simulink model "FlyingBoard_1engine"  (R2018b)
settings: Solver=FixedStepAuto  StartTime=0.0  StopTime=inf  FixedStep=Ts  RelTol=1e-3  EnableMultiTasking=on
values from neighbouring files (symbols this model uses):
  Ts = 1/100    (= 0.01)    [VTOL_params.m]
undefined symbols (not defined in the file or in its folder): dev, Main, pwm_output0
libraries: pwm_sig_converters x5, px4Sensorslib x3, px4uORBlib x3, simulink x2, px4lib x1, aerolibutil x1, sharedtransform x1
settings Model: SimulationMode=external  ExtModeTrigDuration=10  Creator=Robert  LastModifiedBy=Robert
settings SolverCC: PositivePriorityOrder=on
settings DataIOCC: SaveOutput=off  SignalLogging=off  DSMLogging=off  SaveTime=off
settings OptimizationCC: DefaultUnderspecifiedDataType=single  EnhancedBackFolding=on  PassReuseOutputArgsAs=Individual arguments  MaxStackSize=64  OptimizeBlockOrder=speed  DifferentSizesBufferReuse=on  OptimizationCustomize=off
settings DebuggingCC: ParameterTunabilityLossMsg=error
settings HardwareCC: ProdBitPerPointer=32  ProdBitPerSizeT=32  ProdBitPerPtrDiffT=32  ProdLargestAtomicInteger=Long  ProdLargestAtomicFloat=Double  ProdWordSize=32  ProdLongLongMode=on  ProdHWDeviceType=ARM Compatible->ARM Cortex
settings SFSimCC: MATLABDynamicMemAlloc=off
settings RTWCC: SystemTargetFile=ert.tlc  HardwareBoard=PX4 Pixhawk 1  TLCOptions="-aInlineSetEventsForThisBaseRateFcn=TLC_FALSE -aSuppressMultiTaskScheduler=TLC_FALSE  -aRateBasedStepFcn=0"  TemplateMakefile=ert_default_tmf  GenerateReport=on  Toolchain=GNU Tools for PX4 Autopilots  BuildConfiguration=Faster Runs  IncludeHyperlinkInReport=on  LaunchReport=on  TargetLang=C++  GenerateTraceInfo=on  GenerateTraceReport=on  GenerateTraceReportSl=on  GenerateTraceReportSf=on  GenerateTraceReportEml=on
settings CodeAppCC: ForceParamTrailComments=on  IgnoreCustomStorageClasses=off  OperatorAnnotations=on  SimulinkDataObjDesc=on  SFDataObjDesc=on  InsertBlockDesc=on

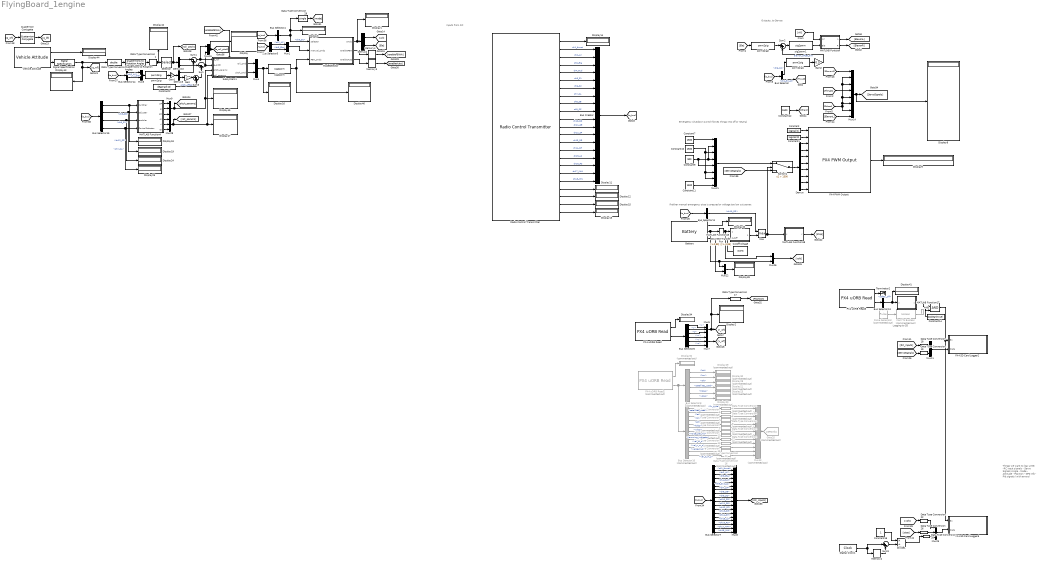
== system FlyingBoard_1engine ==
  note: Emergency shutdown switch forces things into
      | off or neutral
  note: Inputs from RC
  note: Outputs, to Servos
  note: If either manual emergency stop is pressed or voltage too low cut power.
  note: Logging to SD
  note: Things we want to log:
      |
      | uint8
      | -RC input signals
      | - Servo Signals
      |
      | single
      | - Mode
      | - Attitude
      | - Position
      | - GPS info
      | - Pid signals (with errors)
  AND : Logic  IconShape=distinctive  AllPortsSameDT=off  OutDataTypeStr=boolean
  Battery : px4Sensorslib/Battery  voltage=on  current=off  remaining=on  warning=off  timestamp=off  sampleTime=Ts  BlockingMode=off  BlockTimeout=1e-3
      settings: SourceProductName=Embedded Coder Support Package for PX4 Autopilots
  Bus Creator : BusCreator  Inputs=18
  Bus Selector : BusSelector  OutputSignals=ch6_S2,ch1_thrust
  Bus Selector10 : BusSelector  Commented=on  OutputSignals=fix_type,satellites_used,lat,lon,alt,hdop,vdop,noise_per_ms,jamming_indicator,vel_m_s,vel_n_m_s,vel_e_m_s,vel_d_m_s
  Bus Selector11 : BusSelector  OutputSignals=ch10_SD
  Bus Selector13 : BusSelector  OutputSignals=safety_off
  Bus Selector14 : BusSelector  OutputSignals=ch2_Ail,ch3_Ele
  Bus Selector15 : BusSelector  OutputSignals=ch8_SB,ch5_S1,ch12_SF,ch7_SA
  Bus Selector4 : BusSelector  OutputSignals=ch9_SC
  Bus Selector5 : BusSelector  OutputSignals=ch2_Ail,ch3_Ele
  Bus Selector6 : BusSelector  OutputSignals=x,y,z,vx,vy,vz
  Bus Selector7 : BusSelector  OutputSignals=ch1_thrust,ch2_Ail,ch3_Ele,ch4_Rud,ch5_S1,ch6_S2,ch7_SA,ch8_SB,ch9_SC,ch10_SD,ch11_SE,ch12_SF,ch13_SG,ch14_SH,ch15_LS,ch16_RS,ch17_MAX,ch18_MIN
  Bus Selector8 : BusSelector  Commented=on  OutputSignals=lat,lon,alt,satellites_used,hdop,vdop
  Cast To Boolean : DataTypeConversion  Commented=on  OutDataTypeStr=boolean
  Constant : Constant  Value=logical(1)
  Constant1 : Constant  Value=logical(0)
  Constant10 : Constant  Value=1500  OutDataTypeStr=uint16
  Constant11 : Constant  Value=1500  OutDataTypeStr=uint16
  Constant12 : Constant  Value=1500  OutDataTypeStr=uint16  SampleTime=Ts
  Constant14 : Constant  Value=boolean(true)  SampleTime=Ts
  Constant16 : Constant  SampleTime=Ts
  Constant2 : Constant  Value=deg2rad(10)  OutDataTypeStr=single
  Constant7 : Constant  Value=1500  OutDataTypeStr=uint16
  Constant9 : Constant  Value=900  OutDataTypeStr=uint16
  CutoffVoltage : Constant  Value=3.0*3  OutDataTypeStr=single  SampleTime=Ts
  Data Type Conversion : DataTypeConversion  OutDataTypeStr=double
  Data Type Conversion{1,17,22,26,28..29} (6 alike) : DataTypeConversion  OutDataTypeStr=single
  Data Type Conversion{4..16} (13 alike) : DataTypeConversion  Commented=on  OutDataTypeStr=single
  Data Type Conversion18 : DataTypeConversion  OutDataTypeStr=uint16
  Data Type Conversion19 : DataTypeConversion  OutDataTypeStr=uint16
  Demux : Demux  Outputs=8
  Demux10 : Demux  Outputs=2
  Demux2 : Demux  Outputs=2
  Demux3 : Demux  Outputs=2
  Digital Clock1 : DigitalClock  SampleTime=Ts
  Discrete Transfer Fcn : DiscreteTransferFcn  Numerator=[1-0.99]  Denominator=[1 -0.99]  SampleTime=Ts
  Display{,1..3,8..9,11..19,24..25,34,39..46} (26 alike) : Display
      Display9 settings: Format=binary (Stored Integer)
  Display{20..21,23,28..30,32} (7 alike) : Display  Commented=on
  Divide1 : Product  Inputs=*/
  Gain : Gain  Gain=-1
  Gain1 : Gain
  Gain2 : Gain  Gain=0.5
  Goto25 : Goto  Commented=on  GotoTag=GPSinfo
  MATLAB Function : MATLAB Function  TreatAsAtomicUnit=on
  MATLAB Function15 : MATLAB Function  TreatAsAtomicUnit=on
  MATLAB Function17 : MATLAB Function  TreatAsAtomicUnit=on
  MATLAB Function18 : MATLAB Function  TreatAsAtomicUnit=on
  MATLAB Function4 : MATLAB Function  TreatAsAtomicUnit=on
  Max : MinMax  Function=max  Inputs=2  OutDataTypeStr=uint16
  Memory2 : Memory  InheritSampleTime=on
  Memory3 : Memory  InheritSampleTime=on
  Memory4 : Memory  InheritSampleTime=on
  ModeSelector : MATLAB Function  TreatAsAtomicUnit=on
  Mux{1,3..4,11,15,22,26} (7 alike) : Mux  Inputs=2
  Mux13 : Mux  Commented=on  Inputs=13
  Mux14 : Mux  Inputs=8
  Mux21 : Mux  Inputs=8
  Mux{5,7,9,25,28} (5 alike) : Mux  Inputs=3
  Mux8 : Mux  Inputs=18
  PX4 PWM Output : px4lib/PX4 PWM Output  pwmDevice=Main (/dev/pwm_output0)  pwmChannel1_=on  pwmChannel2_=on  pwmChannel3_=on  pwmChannel4_=on  pwmChannel5_=on  pwmChannel6_=on  pwmChannel7_=on  pwmChannel8_=on  forceTerminateFailsafe=off  outputErrorStatus=on
      settings: SourceProductName=Embedded Coder Support Package for PX4 Autopilots
  PX4 SD Card Logger2 : Subsystem  mask(PX4 SD Card Logger){logfile=/fs/microsd/log, logfilename=rc_and_servosignals, cacheflag=off, numRecs=250*60*60}
      mask prompts: logfile "Log Folder"; logfilename "Log File Name"; cacheflag "Cache in Memory"; numRecs "Maximum Record Count"
      mask help:
      | Log data to a specified file on the SD card
      |
      | The block accepts two inputs, enable and data. The incoming data is logged into the SD card when the enable signal is high and the number of data points logged is less than the Maximum Record Count specified.
      |
      | The specified folder should be present in the SD card for logging.
      |
      | If Cache in Memory is unchecked, the data is written to the SD card at every timestep.  If Cache in Memory is checked, data is cached in the memory and is written to SD card only when enable goes low or when the number of data points logged reaches the Maximum Record Count specified.
      mask init:
      | logname=uint8([logfile,'/',logfilename]);
      mask Help: eval('codertarget.internal.helpView(''px4'',''px4sdcardexample'')');
      mask Display:
      | fprintf([get_param(gcb,'logfile'),'/',get_param(gcb,'logfilename')])
      | port_label('input',1,'en')
      | port_label('input',2,'data')
  PX4 SD Card Logger6 : Subsystem  mask(PX4 SD Card Logger){logfile=/fs/microsd/log, logfilename=volt_stop, cacheflag=off, numRecs=250*60*60}
      mask prompts: logfile "Log Folder"; logfilename "Log File Name"; cacheflag "Cache in Memory"; numRecs "Maximum Record Count"
      mask help:
      | Log data to a specified file on the SD card
      |
      | The block accepts two inputs, enable and data. The incoming data is logged into the SD card when the enable signal is high and the number of data points logged is less than the Maximum Record Count specified.
      |
      | The specified folder should be present in the SD card for logging.
      |
      | If Cache in Memory is unchecked, the data is written to the SD card at every timestep.  If Cache in Memory is checked, data is cached in the memory and is written to SD card only when enable goes low or when the number of data points logged reaches the Maximum Record Count specified.
      mask init:
      | logname=uint8([logfile,'/',logfilename]);
      mask Help: eval('codertarget.internal.helpView(''px4'',''px4sdcardexample'')');
      mask Display:
      | fprintf([get_param(gcb,'logfile'),'/',get_param(gcb,'logfilename')])
      | port_label('input',1,'en')
      | port_label('input',2,'data')
  PX4 uORB Read : px4uORBlib/PX4 uORB Read  uORBTopic=vehicle_local_position  sampleTime=Ts  BlockingMode=off  BlockTimeout=1e-3
      settings: SourceProductName=Embedded Coder Support Package for PX4 Autopilots
  PX4 uORB Read2 : px4uORBlib/PX4 uORB Read  Commented=on  uORBTopic=vehicle_gps_position  sampleTime=0.004  BlockingMode=off  BlockTimeout=1e-3
      settings: SourceProductName=Embedded Coder Support Package for PX4 Autopilots
  PX4 uORB Read3 : px4uORBlib/PX4 uORB Read  uORBTopic=safety  sampleTime=Ts  BlockingMode=off  BlockTimeout=1e-3
      settings: SourceProductName=Embedded Coder Support Package for PX4 Autopilots
  Pulse Generator : DiscretePulseGenerator  Commented=on  SampleTime=Ts
  Quaternion Conjugate : aerolibutil/Quaternion Conjugate
      settings: SourceProductName=Aerospace Blockset  SourceProductBaseCode=AE
  Quaternions to Rotation Angles : sharedtransform/Quaternions to Rotation Angles  rotationOrder=ZYX  aMode=aMode
      settings: SourceProductBaseCode=AE
  Radio Control Transmitter : px4Sensorslib/Radio Control Transmitter  channel1=on  channel2=on  channel3=on  channel4=on  channel5=on  channel6=on  channel7=on  channel8=on  channel9=on  channel10=on  channel11=on  channel12=on  channel13=on  channel14=on  channel15=on  channel16=on  channel17=on  channel18=on  channel_count=on  rssi=on  rc_input_source=on  timestamp_last_signal=on  time_stamp=off  sampleTime=Ts  BlockingMode=off  BlockTimeout=5
      settings: SourceProductName=Embedded Coder Support Package for PX4 Autopilots
  Selector : Selector  InputPortWidth=3  IndexOptions=Index vector (dialog)  Indices=[3 2]  OutputSizes=1
  Signal Specification : SignalSpecification  OutDataTypeStr=single
  Subsystem1 : Subsystem
  Sum : Sum  Inputs=|-+
  Sum1 : Sum  Inputs=|-+
  Sum2 : Sum  Inputs=|++
  Sum3 : Sum  Inputs=|++
  Sum9 : Sum  Inputs=|+-
  Switch1 : Switch  Criteria=u2 > Threshold  Threshold=1300
  Terminator2 : Terminator
  Vehicle Attitude : px4Sensorslib/Vehicle Attitude  rollRate=off  pitchRate=off  yawRate=off  quaternion=on  uorbTimeStamp=off  BlockingMode=off  BlockTimeout=0.001  sampleTime=Ts
      settings: SourceProductName=Embedded Coder Support Package for PX4 Autopilots
  pwm2sig : pwm_sig_converters/pwm2sig  SystemSampleTime=-1
  pwm2sig1 : pwm_sig_converters/pwm2sig  SystemSampleTime=-1
  pwm2sig2 : pwm_sig_converters/pwm2sig  SystemSampleTime=-1
  sig2pwm : pwm_sig_converters/sig2pwm  SystemSampleTime=-1
  sig2pwm1 : pwm_sig_converters/sig2pwm  SystemSampleTime=-1
  wires:
  Bus Selector7/10 -> Mux8/10  "<ch10_SD>"
  Battery/3 -> Mux22/2
  [rc_bus] -> Bus Selector11/1
  Switch1/1 -> Demux/1
  Battery/2 -> Discrete Transfer Fcn/1, Mux26/2, Mux22/1
  Demux/8 -> PX4 PWM Output/10
  Data Type Conversion8/1 -> Mux13/5
  Constant11/1 -> Mux21/8
  Radio Control Transmitter/16 -> Bus Creator/15  "ch15_LS"
  Constant7/1 -> Mux21/1
  Demux/1 -> PX4 PWM Output/3
  Constant9/1 -> Mux21/2, Mux21/4, Mux21/5
  Bus Selector7/2 -> Mux8/2  "<ch2_Ail>"
  Radio Control Transmitter/8 -> Bus Creator/7  "ch7_SA"
  [ServoSignals] -> Switch1/3
  Bus Selector10/2 -> Data Type Conversion5/1  "<satellites_used>"
  Max/1 -> MATLAB Function18/1(u), Switch1/2
  Bus Selector7/3 -> Mux8/3  "<ch3_Ele>"
  Bus Selector10/6 -> Data Type Conversion9/1  "<hdop>"
  Data Type Conversion6/1 -> Mux13/3
  Constant10/1 -> Mux21/7, Mux21/6, Mux21/3
  Bus Selector6/5 -> Mux7/2  "<vy>"
  MATLAB Function15/1(stopsig) -> Max/2
  Radio Control Transmitter/19 -> Bus Creator/18  "ch18_MIN"
  Data Type Conversion9/1 -> Mux13/6
  Bus Selector8/4 -> Display21/1  "<satellites_used>"
  Bus Selector10/10 -> Data Type Conversion13/1  "<vel_m_s>"
  Bus Selector6/1 -> Mux5/1  "<x>"
  PX4 PWM Output/1 -> Display9/1
  Mux22/1 -> Display39/1
  Bus Selector11/1 -> Max/1  "<ch10_SD>"
  Radio Control Transmitter/21 -> Display12/1
  Demux/4 -> PX4 PWM Output/6
  Data Type Conversion7/1 -> Mux13/4
  Bus Selector10/9 -> Data Type Conversion12/1  "<jamming_indicator>"
  Demux/3 -> PX4 PWM Output/5
  Bus Selector8/1 -> Display29/1  "<lat>"
  Mux21/1 -> Switch1/1
  Bus Selector7/8 -> Mux8/8  "<ch8_SB>"
  Data Type Conversion16/1 -> Mux13/13
  Radio Control Transmitter/6 -> Bus Creator/5  "ch5_S1"
  [ElevonR] -> Mux14/1
  Bus Selector10/11 -> Data Type Conversion14/1  "<vel_n_m_s>"
  Bus Selector6/4 -> Mux7/1  "<vx>"
  Bus Selector10/8 -> Data Type Conversion11/1  "<noise_per_ms>"
  Data Type Conversion14/1 -> Mux13/11
  Bus Selector10/12 -> Data Type Conversion15/1  "<vel_e_m_s>"
  Bus Selector7/15 -> Mux8/15  "<ch15_LS>"
  Data Type Conversion12/1 -> Mux13/9
  Data Type Conversion13/1 -> Mux13/10
  Bus Selector7/9 -> Mux8/9  "<ch9_SC>"
  Data Type Conversion10/1 -> Mux13/7
  Data Type Conversion5/1 -> Mux13/2
  Demux/6 -> PX4 PWM Output/8
  Demux/7 -> PX4 PWM Output/9
  Mux7/1 -> [v_wf]
  Mux14/1 -> Display8/1, [ServoSignals]
  Bus Selector7/12 -> Mux8/12  "<ch12_SF>"
  Radio Control Transmitter/3 -> Bus Creator/2  "ch2_Ail"
  Bus Selector7/14 -> Mux8/14  "<ch14_SH>"
  Bus Selector7/11 -> Mux8/11  "<ch11_SE>"
  Radio Control Transmitter/23 -> Display13/1
  Bus Selector10/1 -> Data Type Conversion4/1  "<fix_type>"
  [rc_bus] -> Bus Selector7/1
  Bus Selector7/6 -> Mux8/6  "<ch6_S2>"
  Bus Selector10/13 -> Data Type Conversion16/1  "<vel_d_m_s>"
  Bus Selector7/7 -> Mux8/7  "<ch7_SA>"
  Bus Selector7/18 -> Mux8/18  "<ch18_MIN>"
  Data Type Conversion17/1 -> [Position]
  Bus Selector7/4 -> Mux8/4  "<ch4_Rud>"
  Bus Selector7/17 -> Mux8/17  "<ch17_MAX>"
  Radio Control Transmitter/17 -> Bus Creator/16  "ch16_RS"
  Demux/2 -> PX4 PWM Output/4
  Bus Selector7/16 -> Mux8/16  "<ch16_RS>"
  Data Type Conversion11/1 -> Mux13/8
  Radio Control Transmitter/11 -> Bus Creator/10  "ch10_SD"
  Radio Control Transmitter/20 -> Display11/1
  [ElevonL] -> Mux14/8
  PX4 uORB Read/1 -> Display34/1
  [Thrust] -> Mux14/4
  Bus Selector10/4 -> Data Type Conversion7/1  "<lon>"
  Data Type Conversion4/1 -> Mux13/1
  Radio Control Transmitter/14 -> Bus Creator/13  "ch13_SG"
  Bus Selector6/3 -> Mux5/3  "<z>"
  Bus Selector8/2 -> Display30/1  "<lon>"
  PX4 uORB Read/2 -> Bus Selector6/1
  CutoffVoltage/1 -> MATLAB Function15/2(cutoff)
  Radio Control Transmitter/22 -> Display15/1
  Radio Control Transmitter/10 -> Bus Creator/9  "ch9_SC"
  Radio Control Transmitter/15 -> Bus Creator/14  "ch14_SH"
  Radio Control Transmitter/13 -> Bus Creator/12  "ch12_SF"
  Bus Selector7/1 -> Mux8/1  "<ch1_thrust>"
  Radio Control Transmitter/18 -> Bus Creator/17  "ch17_MAX"
  Battery/1 -> Display40/1
  Mux8/1 -> [RC_inputs]
  Bus Selector10/3 -> Data Type Conversion6/1  "<lat>"
  PX4 uORB Read2/1 -> Display32/1
  Radio Control Transmitter/4 -> Bus Creator/3  "ch3_Ele"
  Constant1/1 -> PX4 PWM Output/2
  Bus Creator/1 -> [rc_bus]
  Bus Selector6/6 -> Mux7/3  "<vz>"
  Radio Control Transmitter/5 -> Bus Creator/4  "ch4_Rud"
  Constant/1 -> PX4 PWM Output/1
  Constant12/1 -> [Others]
  Bus Selector7/5 -> Mux8/5  "<ch5_S1>"
  Radio Control Transmitter/1 -> Display14/1
  Radio Control Transmitter/9 -> Bus Creator/8  "ch8_SB"
  PX4 uORB Read2/2 -> Bus Selector10/1, Bus Selector8/1
  Radio Control Transmitter/2 -> Bus Creator/1  "ch1_thrust"
  Bus Selector10/5 -> Data Type Conversion8/1  "<alt>"
  Bus Selector6/2 -> Mux5/2  "<y>"
  Mux13/1 -> Goto25/1
  Radio Control Transmitter/12 -> Bus Creator/11  "ch11_SE"
  Bus Selector7/13 -> Mux8/13  "<ch13_SG>"
  Mux5/1 -> Data Type Conversion17/1, Display2/1, [r_wf]
  Radio Control Transmitter/7 -> Bus Creator/6  "ch6_S2"
  Bus Selector10/7 -> Data Type Conversion10/1  "<vdop>"
  Data Type Conversion15/1 -> Mux13/12
  Bus Selector8/5 -> Display23/1  "<hdop>"
  Demux/5 -> PX4 PWM Output/7
  Bus Selector8/3 -> Display28/1  "<alt>"
  Bus Selector8/6 -> Display20/1  "<vdop>"
  PX4 uORB Read3/2 -> Bus Selector13/1
  Bus Selector13/1 -> MATLAB Function17/1(u), Display41/1  "<safety_off>"
  MATLAB Function17/1(y) -> AND/1
  [RC_inputs] -> Data Type Conversion18/1
  [ServoSignals] -> Data Type Conversion19/1
  Data Type Conversion18/1 -> Mux11/1
  Data Type Conversion19/1 -> Mux11/2
  Mux11/1 -> PX4 SD Card Logger2/2(Data)
  Pulse Generator/1 -> Cast To Boolean/1
  Cast To Boolean/1 -> ?
  Mux25/1 -> PX4 SD Card Logger6/2(Data)
  Data Type Conversion26/1 -> Mux25/2
  AND/1 -> PX4 SD Card Logger6/1(En), PX4 SD Card Logger2/1(En)
  [stop] -> Data Type Conversion26/1
  Data Type Conversion22/1 -> Mux25/1
  [volt] -> Data Type Conversion22/1
  MATLAB Function18/1(y) -> [stop]
  PX4 uORB Read3/1 -> Terminator2/1
  Discrete Transfer Fcn/1 -> MATLAB Function15/1(voltage), Mux26/1
  Mux26/1 -> [volt]
  Constant14/1 -> AND/2
  Divide1/1 -> Data Type Conversion28/1
  Sum9/1 -> Divide1/2
  Constant16/1 -> Divide1/1
  Memory2/1 -> Sum9/2
  Digital Clock1/1 -> Sum9/1, Memory2/1
  Data Type Conversion28/1 -> Mux25/3
  ModeSelector/2(enableFBW) -> Memory4/1
  Memory4/1 -> [enableFBWA]
  Demux10/2 -> Sum/1
  Subsystem1/2(pitch_cmd) -> Mux4/2
  Data Type Conversion29/1 -> [mode]
  Bus Selector15/4 -> Display25/1, MATLAB Function4/4(ControlSelector)  "<ch7_SA>"
  sig2pwm/1 -> ModeSelector/3(FBW_cmds), Display46/1
  Sum1/1 -> Mux15/1, Subsystem1/1(e_roll)
  Demux2/2 -> [Ele]
  Mux15/1 -> Display/1, [e_roll_pitch]
  MATLAB Function4/4(rP) -> Mux28/1
  [q_wf] -> Quaternion Conjugate/1
  ModeSelector/1(cmds) -> Display1/1, Demux2/1
  Memory3/1 -> [enableAuto]
  Bus Selector15/1 -> Display18/1, MATLAB Function4/1(switcher)  "<ch8_SB>"
  pwm2sig/1 -> Gain1/1
  ModeSelector/3(enableAuto) -> Memory3/1
  Mux9/1 -> [pitch_params], Subsystem1/3(pitch_params), Display45/1
  [enableFBWA] -> Subsystem1/Enable
  [rc_bus] -> Bus Selector4/1
  Signal Specification/1 -> [q_wf], Display43/1, Data Type Conversion/1
  MATLAB Function4/3(pD) -> Mux9/3
  Demux10/1 -> Sum1/1
  [rc_bus] -> Bus Selector5/1
  Mux4/1 -> sig2pwm/1, Display16/1
  Mux3/1 -> pwm2sig/1
  [rc_bus] -> Bus Selector15/1
  Bus Selector4/1 -> ModeSelector/1(selector), Display3/1, Data Type Conversion29/1  "<ch9_SC>"
  Data Type Conversion/1 -> Quaternions to Rotation Angles/1
  MATLAB Function4/2(pI) -> Mux9/2
  Demux3/2 -> Gain/1
  [rc_bus] -> Bus Selector14/1
  Mux1/1 -> ModeSelector/2(manual_cmds)
  Data Type Conversion1/1 -> Display42/1, Selector/1
  Bus Selector15/3 -> Display24/1, MATLAB Function4/3(enabler)  "<ch12_SF>"
  Demux2/1 -> [Ail]
  Sum/1 -> Subsystem1/2(e_pitch), Mux15/2
  MATLAB Function4/5(rI) -> Mux28/2
  Bus Selector14/2 -> Mux3/2  "<ch3_Ele>"
  Quaternion Conjugate/1 -> [q_bf]
  MATLAB Function4/6(rD) -> Mux28/3
  Quaternions to Rotation Angles/1 -> Data Type Conversion1/1
  Mux28/1 -> [roll_params], Subsystem1/4(roll_params), Display17/1
  Bus Selector5/2 -> Mux1/2  "<ch3_Ele>"
  Vehicle Attitude/2 -> Signal Specification/1
  Vehicle Attitude/1 -> Display44/1
  Bus Selector14/1 -> Mux3/1  "<ch2_Ail>"
  Bus Selector5/1 -> Mux1/1  "<ch2_Ail>"
  Subsystem1/1(roll_cmd) -> Mux4/1
  Bus Selector15/2 -> Display19/1, MATLAB Function4/2(adjuster)  "<ch5_S1>"
  MATLAB Function4/1(pP) -> Mux9/1
  Selector/1 -> [roll_pitch], Demux10/1
  [Others] -> Mux14/5, Mux14/2, Mux14/3, Mux14/6, Mux14/7
  [Ail] -> MATLAB Function/1(Ail)
  Sum2/1 -> sig2pwm1/1
  MATLAB Function/2(R) -> [ElevonR]
  MATLAB Function/1(L) -> [ElevonL]
  [rc_bus] -> Bus Selector/1
  Bus Selector/2 -> [Thrust]  "<ch1_thrust>"
  Sum3/1 -> Sum/2
  Demux3/1 -> Sum1/2
  Gain1/1 -> Demux3/1
  [Ele] -> pwm2sig2/1
  Bus Selector/1 -> pwm2sig1/1  "<ch6_S2>"
  pwm2sig1/1 -> Gain2/1
  Gain2/1 -> Sum2/2  "elevon_offset_trim"
  pwm2sig2/1 -> Sum2/1
  sig2pwm1/1 -> MATLAB Function/2(Ele)
  Gain/1 -> Sum3/1
  Constant2/1 -> Sum3/2  "pitch_offset"

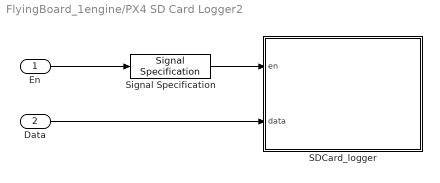
== system FlyingBoard_1engine/PX4 SD Card Logger2 ==
  En : Inport
  Data : Inport  Port=2
  SDCard_logger : MATLAB Function  TreatAsAtomicUnit=on
  Signal Specification : SignalSpecification  OutDataTypeStr=boolean
  wires:
  Signal Specification/1 -> SDCard_logger/1(en)
  En/1 -> Signal Specification/1
  Data/1 -> SDCard_logger/2(data)

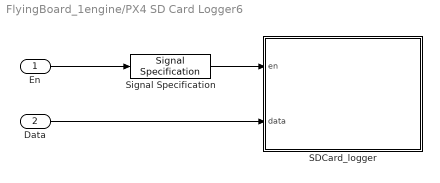
== system FlyingBoard_1engine/PX4 SD Card Logger6 ==
  En : Inport
  Data : Inport  Port=2
  SDCard_logger : MATLAB Function  TreatAsAtomicUnit=on
  Signal Specification : SignalSpecification  OutDataTypeStr=boolean
  wires:
  Signal Specification/1 -> SDCard_logger/1(en)
  En/1 -> Signal Specification/1
  Data/1 -> SDCard_logger/2(data)

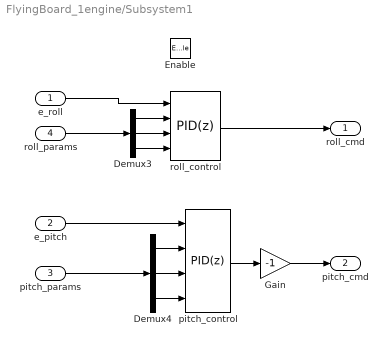
== system FlyingBoard_1engine/Subsystem1 ==
  e_roll : Inport
  e_pitch : Inport  Port=2
  pitch_params : Inport  Port=3
  roll_params : Inport  Port=4
  Enable : EnablePort
  Demux3 : Demux  Outputs=3
  Demux4 : Demux  Outputs=3
  Gain : Gain  Gain=-1
  pitch_control : simulink/Continuous/PID Controller  Controller=PID  Form=Parallel  TimeDomain=Discrete-time  SampleTime=Ts  IntegratorMethod=Backward Euler  FilterMethod=Forward Euler  ControllerParametersSource=external  P=1  I=0  D=0  UseFilter=off  N=100  TunerSelectOption=Transfer Function Based (PID Tuner App)  InitialConditionSource=internal  InitialConditionForIntegrator=0  InitialConditionForFilter=0  DifferentiatorICPrevScaledInput=0  ExternalReset=none  TrackingMode=off  Kt=1  LimitOutput=on  UpperSaturationLimit=1  LowerSaturationLimit=-1  LinearizeAsGain=off  AntiWindupMode=clamping  Kb=1  PGainOutDataTypeStr=single  PProdOutDataTypeStr=single  POutMin=[]  POutMax=[]  IGainOutDataTypeStr=single  IProdOutDataTypeStr=single  IOutMin=[]  IOutMax=[]  DGainOutDataTypeStr=single  DProdOutDataTypeStr=single  DOutMin=[]  DOutMax=[]  NOutMin=[]  NOutMax=[]  SumOutDataTypeStr=single  SumOutMin=[]  SumOutMax=[]  SaturationOutDataTypeStr=single  SaturationOutMin=[]  SaturationOutMax=[]  PParamDataTypeStr=single  PParamMin=[]  PParamMax=[]  IParamDataTypeStr=single  IParamMin=[]  IParamMax=[]  DParamDataTypeStr=single  DParamMin=[]  DParamMax=[]  NParamMin=[]  NParamMax=[]  KbParamMin=[]  KbParamMax=[]  KtParamMin=[]  KtParamMax=[]  KbOutMin=[]  KbOutMax=[]  KtOutMin=[]  KtOutMax=[]  IntegratorOutDataTypeStr=single  IntegratorOutMin=[]  IntegratorOutMax=[]  FilterOutMin=[]  FilterOutMax=[]  SumI1OutMin=[]  SumI1OutMax=[]  SumI2OutMin=[]  SumI2OutMax=[]  SumI3OutMin=[]  SumI3OutMax=[]  SumI4OutMin=[]  SumI4OutMax=[]  SumDOutMin=[]  SumDOutMax=[]  SumAccumDataTypeStr=single  DifferentiatorOutDataTypeStr=single  DifferentiatorOutMin=[]  DifferentiatorOutMax=[]  FilterDiffOutCoefMin=[]  FilterDiffOutCoefMax=[]  ReciprocalOutMin=[]  ReciprocalOutMax=[]  SumDenOutMin=[]  SumDenOutMax=[]  SumNumOutMin=[]  SumNumOutMax=[]  DivideOutMin=[]  DivideOutMax=[]  IntegratorContinuousStateAttributes=''  IntegratorStateMustResolveToSignalObject=off  IntegratorRTWStateStorageClass=Auto  FilterContinuousStateAttributes=''  FilterStateMustResolveToSignalObject=off  FilterRTWStateStorageClass=Auto  ParallelPVariant=ExternalParameters  IdealPVariant=Disabled  IVariant=ExternalParameters  DVariant=ExternalParameters  IntegratorVariant=Discrete  SatVariant=Enabled  AWVariant=DiscClampingParallel  PCopyVariant=Disabled  TRVariant=Disabled  FdbkBlocksVariant=Feedback  IdealPFdbkVariant=Passthrough  SatFdbkVariant=Passthrough  DerivativeFilterVariant=Differentiator  NVariant=Passthrough  NCopyVariant=Disabled_SignalSpec  FilterICVariant=InternalICsDifferentiator  IntegratorICVariant=InternalICs  ExternalResetVariant=Disabled  TRSumVariant=Passthrough  SumFdbkVariant=Enabled  SumVariant=Sum_PID
  roll_control : simulink/Continuous/PID Controller  Controller=PID  Form=Parallel  TimeDomain=Discrete-time  SampleTime=Ts  IntegratorMethod=Backward Euler  FilterMethod=Forward Euler  ControllerParametersSource=external  P=1  I=0  D=0  UseFilter=off  N=100  TunerSelectOption=Transfer Function Based (PID Tuner App)  InitialConditionSource=internal  InitialConditionForIntegrator=0  InitialConditionForFilter=0  DifferentiatorICPrevScaledInput=0  ExternalReset=none  TrackingMode=off  Kt=1  LimitOutput=on  UpperSaturationLimit=1  LowerSaturationLimit=-1  LinearizeAsGain=off  AntiWindupMode=clamping  Kb=1  PGainOutDataTypeStr=single  PProdOutDataTypeStr=single  POutMin=[]  POutMax=[]  IGainOutDataTypeStr=single  IProdOutDataTypeStr=single  IOutMin=[]  IOutMax=[]  DGainOutDataTypeStr=single  DProdOutDataTypeStr=single  DOutMin=[]  DOutMax=[]  NOutMin=[]  NOutMax=[]  SumOutDataTypeStr=single  SumOutMin=[]  SumOutMax=[]  SaturationOutDataTypeStr=single  SaturationOutMin=[]  SaturationOutMax=[]  PParamDataTypeStr=single  PParamMin=[]  PParamMax=[]  IParamDataTypeStr=single  IParamMin=[]  IParamMax=[]  DParamDataTypeStr=single  DParamMin=[]  DParamMax=[]  NParamMin=[]  NParamMax=[]  KbParamMin=[]  KbParamMax=[]  KtParamMin=[]  KtParamMax=[]  KbOutMin=[]  KbOutMax=[]  KtOutMin=[]  KtOutMax=[]  IntegratorOutDataTypeStr=single  IntegratorOutMin=[]  IntegratorOutMax=[]  FilterOutMin=[]  FilterOutMax=[]  SumI1OutMin=[]  SumI1OutMax=[]  SumI2OutMin=[]  SumI2OutMax=[]  SumI3OutMin=[]  SumI3OutMax=[]  SumI4OutMin=[]  SumI4OutMax=[]  SumDOutMin=[]  SumDOutMax=[]  SumAccumDataTypeStr=single  DifferentiatorOutDataTypeStr=single  DifferentiatorOutMin=[]  DifferentiatorOutMax=[]  FilterDiffOutCoefMin=[]  FilterDiffOutCoefMax=[]  ReciprocalOutMin=[]  ReciprocalOutMax=[]  SumDenOutMin=[]  SumDenOutMax=[]  SumNumOutMin=[]  SumNumOutMax=[]  DivideOutMin=[]  DivideOutMax=[]  IntegratorContinuousStateAttributes=''  IntegratorStateMustResolveToSignalObject=off  IntegratorRTWStateStorageClass=Auto  FilterContinuousStateAttributes=''  FilterStateMustResolveToSignalObject=off  FilterRTWStateStorageClass=Auto  ParallelPVariant=ExternalParameters  IdealPVariant=Disabled  IVariant=ExternalParameters  DVariant=ExternalParameters  IntegratorVariant=Discrete  SatVariant=Enabled  AWVariant=DiscClampingParallel  PCopyVariant=Disabled  TRVariant=Disabled  FdbkBlocksVariant=Feedback  IdealPFdbkVariant=Passthrough  SatFdbkVariant=Passthrough  DerivativeFilterVariant=Differentiator  NVariant=Passthrough  NCopyVariant=Disabled_SignalSpec  FilterICVariant=InternalICsDifferentiator  IntegratorICVariant=InternalICs  ExternalResetVariant=Disabled  TRSumVariant=Passthrough  SumFdbkVariant=Enabled  SumVariant=Sum_PID
  roll_cmd : Outport
  pitch_cmd : Outport  Port=2
  wires:
  roll_control/1 -> roll_cmd/1
  Demux4/3 -> pitch_control/4
  Demux4/2 -> pitch_control/3
  Demux4/1 -> pitch_control/2
  pitch_params/1 -> Demux4/1
  Demux3/3 -> roll_control/4
  Demux3/2 -> roll_control/3
  Demux3/1 -> roll_control/2
  pitch_control/1 -> Gain/1
  e_roll/1 -> roll_control/1
  e_pitch/1 -> pitch_control/1
  roll_params/1 -> Demux3/1
  Gain/1 -> pitch_cmd/1

== matlab function FlyingBoard_1engine/MATLAB Function ==
  data: Ail input; L output; Ele input; R output
function [L,R] = fcn(Ail,Ele)

A = single(Ail);
E = single(Ele);
L = uint16( -(A-1500)-(E-1500) +1500 );
R = uint16( -(A-1500)+(E-1500) +1500 );

L = min(uint16(2100),L);
R = min(uint16(2100),R);

L = max(uint16(900),L);
R = max(uint16(900),R);

== matlab function FlyingBoard_1engine/MATLAB Function4 ==
  data: switcher input uint16; pP output single; adjuster input uint16; pI output single; pD output single; enabler input uint16; ControlSelector input uint16; rP output single; rI output single; rD output single
function [pP,pI,pD,rP,rI,rD] = fcn(switcher, adjuster, enabler, ControlSelector)

init_params = single(1.5.*[0.5,0,0.01;0.5,0,0.01]); % Pitch;roll

persistent pkP pkI pkD rkP rkI rkD;
if isempty(pkP)
    % OScillation time was 0.25 seconds at P=1, D = 0.025, roll was D=0.05
    pkP = init_params(1,1);
end
if isempty(pkI)
    pkI = init_params(1,2);
end
if isempty(pkD)
    pkD = init_params(1,3);
end
if isempty(rkP)
    rkP = init_params(2,1);
end
if isempty(rkI)
    rkI = init_params(2,2);
end
if isempty(rkD)
    rkD = init_params(2,3);
end

% Below we allow adjustments to be made in the rand [0,2*init_val] (roughly).
% If integrators are set to zero they cannot be enabled by adjusting.
if enabler>1500
    if ControlSelector < 1400 % Top, Roll controll
        if switcher < 1400 % Top, P
            rkP = init_params(2,1)+init_params(2,1)*(single(adjuster)-1500)./500; 
        elseif switcher > 1600 % Bottom, D
            rkD = init_params(2,3)+init_params(2,3)*(single(adjuster)-1500)./500;
        else
            rkI = init_params(2,2)+init_params(2,2)*(single(adjuster)-1500)./500;
        end
    elseif ControlSelector < 1600 % Mid, Pitch control
        if switcher < 1400 % Top, P
            pkP = init_params(1,1)+init_params(1,1)*(single(adjuster)-1500)./500; 
        elseif switcher > 1600 % Bottom, D
            pkD = init_params(1,3)+init_params(1,3)*(single(adjuster)-1500)./500;
        else
            pkI = init_params(1,2)+init_params(1,2)*(single(adjuster)-1500)./500;
        end
    else
        % No controller set here yet
    end
end

pP = pkP;
pI = pkI;
pD = pkD;
rP = rkP;
rI = rkI;
rD = rkD;

== matlab function FlyingBoard_1engine/ModeSelector ==
  data: selector input uint16; cmds output uint16 size=[2,1]; manual_cmds input uint16; FBW_cmds input uint16; enableFBW output boolean; enableAuto output
function [cmds,enableFBW,enableAuto] = fcn(selector, manual_cmds, FBW_cmds)

if selector>1400 % Auto mode, stick down on remote
    cmds = FBW_cmds;
    enableFBW = true;
    enableAuto = false;
else
    cmds = manual_cmds; % As midpoint, but less pitch sensitive.
    enableFBW = false;
    enableAuto = false;
end

== matlab function FlyingBoard_1engine/PX4 SD Card Logger2/SDCard_logger ==
  data: en input boolean; data input; logname parameter uint8; cacheflag parameter boolean; numRecs parameter uint32
%% PX4 SD Card Logger
% Note: All data needs to be of the same type (e.g. double)
% Header information format:
%           String "MWLOG"
%           Time/Date 4 bytes (time())
%           Number of Signals per record Logged 1 byte (256 max)
%           Data Type of Signals Logged  1 byte (1-10)
%           Number of bytes per record 2 bytes (65535 max)
% This does NOT include the number of data sets logged.
% i.e. The Reader is responsible for reading until EOF.
% Steve Kuznicki
% Copyright 2018 The MathWorks, Inc.

function SDCard_logger(en, data, logname, cacheflag, numRecs)

persistent fp count elem_size vect_size datastore timestore count_prev

if coder.target('Rtw')
    
    coder.cinclude('<stdio.h>');
    coder.cinclude('<time.h>');
    
    if coder.target('Rtw')
        coder.cinclude('<drivers/drv_hrt.h>');
    end
    
    if coder.target('Rtw')
        timestamp=coder.opaque('uint64_t');
        timestamp=coder.ceval('hrt_absolute_time');
    else
        timestamp = uint64(0);
    end
    
    if isempty(count)
        count = uint32(0);
        count_prev=count;
        fp = coder.opaque('FILE*', 'NULL');
        if cacheflag == true
            datastore = zeros(numRecs*uint32(coder.const(numel(data))), 1, 'like', data);
            timestore=uint64(zeros(numRecs, 1));
        end
        
        [elsize, eltype] = get_elem_size(data);
        elem_size = coder.const(uint16(elsize));
        elem_type = coder.const(uint8(eltype));
        vect_size = coder.const(uint8(numel(data)));
        coder.ceval('printf',['OPENING file %s vect_size %d elem_size %d numRecs %d %c' uint8(0)], ...
            [logname,'.bin', int8(0)], uint32(vect_size), uint32(elem_size), uint32(numRecs), uint8(10));
        fp = coder.ceval('fopen', [logname,'.bin', int8(0)], ['wb', int8(0)]);
        
        % Write header information here
        % header token + version
        mlStrVer = 'MWLOG';
        coder.ceval('fwrite', coder.rref(mlStrVer), uint32(1), length(mlStrVer), fp);
        % date/time
        tm = uint32(0);
        tmptr = uint32(0);
        tm = coder.ceval('time',coder.wref(tmptr));
        coder.ceval('fwrite', coder.rref(tm), uint32(4), uint32(1), fp);
        % number of elements in each record
        coder.ceval('fwrite', coder.rref(vect_size), uint32(1), uint32(1), fp);
        % data type of the elements
        coder.ceval('fwrite', coder.rref(elem_type), uint32(1), uint32(1), fp);
        % size of each record in bytes
        recSize = elem_size * uint16(vect_size);
        coder.ceval('fwrite', coder.rref(recSize), uint32(2), uint32(1), fp);
        coder.ceval('fclose', fp);
    end
    
    
    if (en && (count < numRecs))
              
        % cache data in memory or use fwrite
        if cacheflag == true
            addr = (count*uint32(vect_size))+1;
            for idx = 1:vect_size
                datastore(addr) = data(idx);
                addr = addr + 1;
            end
            timestore(count+uint32(1))=uint64(timestamp);
        else
            % open file in append mode
            fp = coder.ceval('fopen', [logname,'.bin', int8(0)], ['ab', int8(0)]);
            coder.ceval('fwrite', coder.rref(data), elem_size, vect_size, fp);
            if coder.target('Rtw')
                coder.ceval('fwrite', coder.rref(timestamp), uint32(8), uint32(1), fp);
            end
            coder.ceval('fflush', fp);
            coder.ceval('fclose', fp);
        end
        count = count + uint32(1);
        
    else
        % open file in append mode
        fp = coder.ceval('fopen', [logname,'.bin', int8(0)], ['ab', int8(0)]);            
        coder.ceval('printf',['CLOSING file. count = %d %c' uint8(0)], uint32(count), uint8(10));
        if cacheflag
            for idx=count_prev+1:count
                for idx2=(idx-1)*double(vect_size)+1:(idx-1)*double(vect_size)+double(vect_size)
                    coder.ceval('fwrite', coder.rref(datastore(idx2)), elem_size, uint32(1), fp);
                end
                coder.ceval('fwrite', coder.rref(timestore(idx)), uint32(8), uint32(1), fp);
            end
        end
        coder.ceval('fflush', fp);
        coder.ceval('fclose', fp);
        count_prev=count;
    end
end

% return the size of the element in bytes
    function [elem_size, dtype] = get_elem_size(data)
        switch(class(data))
            case 'double'
                elem_size = 8;
                dtype = 1;
            case 'single'
                elem_size = 4;
                dtype = 2;
            case 'int32'
                elem_size = 4;
                dtype = 3;
            case 'uint32'
                elem_size = 4;
                dtype = 4;
            case 'int16'
                elem_size = 2;
                dtype = 5;
            case 'uint16'
                elem_size = 2;
                dtype = 6;
            case 'int8'
                elem_size = 1;
                dtype = 7;
            case 'uint8'
                elem_size = 1;
                dtype = 8;
            case 'logical'
                elem_size = 1;
                dtype = 9;
            case 'embedded.fi'
                nt = numerictype(data);
                elem_size = 2^ceil(log2(ceil(nt.WordLength / 8)));
                dtype = 10;
        end
        if ~isreal(data)
            elem_size = elem_size*2;
        end
        
        elem_size = uint16(elem_size);
        dtype = uint8(dtype);
    end
end

== matlab function FlyingBoard_1engine/MATLAB Function15 ==
  data: voltage input single; stopsig output uint16; cutoff input single
function stopsig = fcn(voltage, cutoff)

if voltage<cutoff
    stopsig = uint16(2000);
else
    stopsig = uint16(1000);
end

== matlab function FlyingBoard_1engine/MATLAB Function17 ==
  data: u input; y output
function y = logstarter(u)
%At first arm, start logging and dont quit

persistent state;

if isempty(state)
    state = 0;
end

if u>0
    state = 1;
end

y = state;

== matlab function FlyingBoard_1engine/PX4 SD Card Logger6/SDCard_logger ==
  data: en input boolean; data input; logname parameter uint8; cacheflag parameter boolean; numRecs parameter uint32
%% PX4 SD Card Logger
% Note: All data needs to be of the same type (e.g. double)
% Header information format:
%           String "MWLOG"
%           Time/Date 4 bytes (time())
%           Number of Signals per record Logged 1 byte (256 max)
%           Data Type of Signals Logged  1 byte (1-10)
%           Number of bytes per record 2 bytes (65535 max)
% This does NOT include the number of data sets logged.
% i.e. The Reader is responsible for reading until EOF.
% Steve Kuznicki
% Copyright 2018 The MathWorks, Inc.

function SDCard_logger(en, data, logname, cacheflag, numRecs)

persistent fp count elem_size vect_size datastore timestore count_prev

if coder.target('Rtw')
    
    coder.cinclude('<stdio.h>');
    coder.cinclude('<time.h>');
    
    if coder.target('Rtw')
        coder.cinclude('<drivers/drv_hrt.h>');
    end
    
    if coder.target('Rtw')
        timestamp=coder.opaque('uint64_t');
        timestamp=coder.ceval('hrt_absolute_time');
    else
        timestamp = uint64(0);
    end
    
    if isempty(count)
        count = uint32(0);
        count_prev=count;
        fp = coder.opaque('FILE*', 'NULL');
        if cacheflag == true
            datastore = zeros(numRecs*uint32(coder.const(numel(data))), 1, 'like', data);
            timestore=uint64(zeros(numRecs, 1));
        end
        
        [elsize, eltype] = get_elem_size(data);
        elem_size = coder.const(uint16(elsize));
        elem_type = coder.const(uint8(eltype));
        vect_size = coder.const(uint8(numel(data)));
        coder.ceval('printf',['OPENING file %s vect_size %d elem_size %d numRecs %d %c' uint8(0)], ...
            [logname,'.bin', int8(0)], uint32(vect_size), uint32(elem_size), uint32(numRecs), uint8(10));
        fp = coder.ceval('fopen', [logname,'.bin', int8(0)], ['wb', int8(0)]);
        
        % Write header information here
        % header token + version
        mlStrVer = 'MWLOG';
        coder.ceval('fwrite', coder.rref(mlStrVer), uint32(1), length(mlStrVer), fp);
        % date/time
        tm = uint32(0);
        tmptr = uint32(0);
        tm = coder.ceval('time',coder.wref(tmptr));
        coder.ceval('fwrite', coder.rref(tm), uint32(4), uint32(1), fp);
        % number of elements in each record
        coder.ceval('fwrite', coder.rref(vect_size), uint32(1), uint32(1), fp);
        % data type of the elements
        coder.ceval('fwrite', coder.rref(elem_type), uint32(1), uint32(1), fp);
        % size of each record in bytes
        recSize = elem_size * uint16(vect_size);
        coder.ceval('fwrite', coder.rref(recSize), uint32(2), uint32(1), fp);
        coder.ceval('fclose', fp);
    end
    
    
    if (en && (count < numRecs))
              
        % cache data in memory or use fwrite
        if cacheflag == true
            addr = (count*uint32(vect_size))+1;
            for idx = 1:vect_size
                datastore(addr) = data(idx);
                addr = addr + 1;
            end
            timestore(count+uint32(1))=uint64(timestamp);
        else
            % open file in append mode
            fp = coder.ceval('fopen', [logname,'.bin', int8(0)], ['ab', int8(0)]);
            coder.ceval('fwrite', coder.rref(data), elem_size, vect_size, fp);
            if coder.target('Rtw')
                coder.ceval('fwrite', coder.rref(timestamp), uint32(8), uint32(1), fp);
            end
            coder.ceval('fflush', fp);
            coder.ceval('fclose', fp);
        end
        count = count + uint32(1);
        
    else
        % open file in append mode
        fp = coder.ceval('fopen', [logname,'.bin', int8(0)], ['ab', int8(0)]);            
        coder.ceval('printf',['CLOSING file. count = %d %c' uint8(0)], uint32(count), uint8(10));
        if cacheflag
            for idx=count_prev+1:count
                for idx2=(idx-1)*double(vect_size)+1:(idx-1)*double(vect_size)+double(vect_size)
                    coder.ceval('fwrite', coder.rref(datastore(idx2)), elem_size, uint32(1), fp);
                end
                coder.ceval('fwrite', coder.rref(timestore(idx)), uint32(8), uint32(1), fp);
            end
        end
        coder.ceval('fflush', fp);
        coder.ceval('fclose', fp);
        count_prev=count;
    end
end

% return the size of the element in bytes
    function [elem_size, dtype] = get_elem_size(data)
        switch(class(data))
            case 'double'
                elem_size = 8;
                dtype = 1;
            case 'single'
                elem_size = 4;
                dtype = 2;
            case 'int32'
                elem_size = 4;
                dtype = 3;
            case 'uint32'
                elem_size = 4;
                dtype = 4;
            case 'int16'
                elem_size = 2;
                dtype = 5;
            case 'uint16'
                elem_size = 2;
                dtype = 6;
            case 'int8'
                elem_size = 1;
                dtype = 7;
            case 'uint8'
                elem_size = 1;
                dtype = 8;
            case 'logical'
                elem_size = 1;
                dtype = 9;
            case 'embedded.fi'
                nt = numerictype(data);
                elem_size = 2^ceil(log2(ceil(nt.WordLength / 8)));
                dtype = 10;
        end
        if ~isreal(data)
            elem_size = elem_size*2;
        end
        
        elem_size = uint16(elem_size);
        dtype = uint8(dtype);
    end
end

== matlab function FlyingBoard_1engine/MATLAB Function18 ==
  data: u input; y output
function y = fcn(u)

if u>uint16(1300)
    y = logical(true);
else
    y = logical(false);
end
